simulink model "PlusControllerElegantFix"  (R2021a)
settings: Solver=VariableStepAuto  StartTime=0.0  StopTime=25  RelTol=1e-3
settings Model: Creator=phill  LastModifiedBy=phill

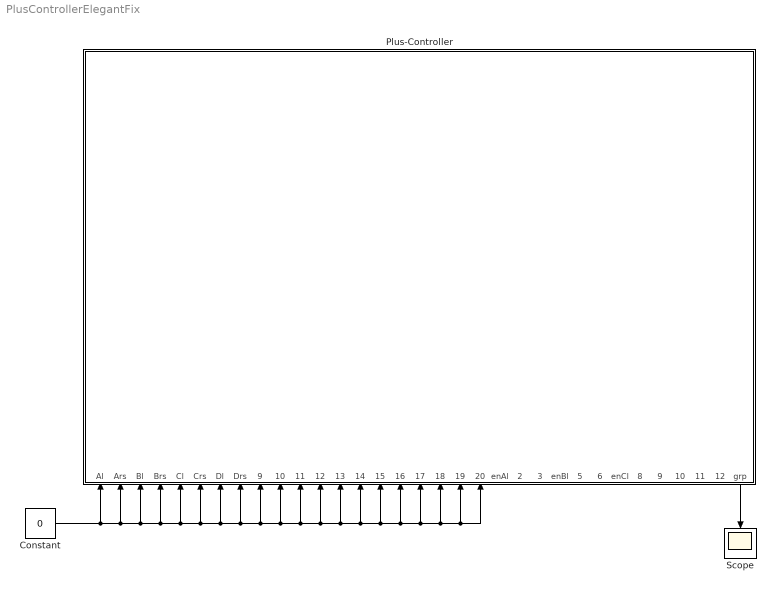
== system PlusControllerElegantFix ==
  Constant : Constant  Value=0
  Plus-Controller : Stateflow chart  TreatAsAtomicUnit=on  mask{green_duration_sr=6, green_duration_l=6, tol=0}
      mask prompts: green_duration_sr "Green Duration for straight/right traffic"; green_duration_l "Green Duration for left traffic"; tol "tolerance"
      settings: PortSchema="{\"entries\":[{\"content\":{\"sides\":[{\"content\":{\"connectorIds\":[]},\"type\":\"ConnectorPlacement.EquallySpacedRectSide\",\"uuid\":\"2590cc03-86a2-4387-8b1b-fdf4c8b68aa6\"},{\"content\":{\"connectorIds\":[],\"side\":\"RIGHT\"},\"type\":\"ConnectorPlacement.EquallySpacedRectSide\",\"uuid\":\"b97063cd-dd31-425f-b4aa-3aaa013ac411\"},{\"content\":{\"connectorIds\":[],\"side\":\"TOP\"},\"type\":\"ConnectorPlacement.EquallySpacedRectSide\",\"uuid\":\"ef5846b9-436e-4b10-a854-1305521b6a0d\"},{\"content\":{\"connectorIds\":[\"In3\",\"In4\",\"In1\",\"In2\",\"In5\",\"In6\",\"In7\",\"In8\",\"In9\",\"In10\",\"In11\",\"In12\",\"In13\",\"In14\",\"In15\",\"In16\",\"In17\",\"In18\",\"In19\",\"In20\",\"Out1\",\"Out2\",\"Out3\",\"Out4\",\"Out5\",\"Out6\",\"Out7\",\"Out8\",\"Out9\",\"Out10\",\"Out11\",\"Out12\",\"Out13\"],\"side\":\"BOTTOM\"},\"type\":\"ConnectorPlacement.EquallySpacedRectSide\",\"uuid\":\"44b73820-3b7c-4ee5-b5da-9465e85a924e\"}]},\"type\":\"ConnectorPlacement.EquallySpacedConnector\",\"uuid\":\"3342797d-7762-4a2a-891a-654024402a66\"}],\"packageUris\":[\"http://schema.mathworks.com/mf0/Connector/R2020b\"],\"version\":\"1.0\"}"
  Scope : Scope
  wires:
  Constant/1 -> Plus-Controller/20(Drs_Bo), Plus-Controller/19(Drs_Ao), Plus-Controller/18(Dl_Co), Plus-Controller/17(Crs_Do), Plus-Controller/16(Crs_Bo), Plus-Controller/15(Cl_Ao), Plus-Controller/14(Brs_Ao), Plus-Controller/13(Brs_Co), Plus-Controller/12(Bl_Do), Plus-Controller/11(Ars_Co), Plus-Controller/10(Ars_Do), Plus-Controller/9(Al_Bo), Plus-Controller/8(Drs), Plus-Controller/7(Dl), Plus-Controller/6(Crs), Plus-Controller/5(Cl), Plus-Controller/2(Brs), Plus-Controller/1(Bl), Plus-Controller/4(Ars), Plus-Controller/3(Al)
  Plus-Controller/13(grp) -> Scope/1

== stateflow chart PlusControllerElegantFix/Plus-Controller ==
  state Group__Crs_Brs
    state init
    note: check
        | Crs straight
        | crossings
    note: check
        | Crs right
        | crossings
    note: check
        | Brs straight
        | crossings
    note: check
        | Brs right
        | crossings
    (default) -> Group__Crs_Brs.init
    (junction 109) -> Group__Crs_Brs.init
    Group__Crs_Brs.init -> (junction 51)
    (junction 51) -> (junction 59) [order 1] : [(Dl_Co<=tol && Drs_Ao<=tol ...
        | && Drs_Bo<=tol && Bl_Do<=tol ...
        | && Al_Bo<=tol && Ars_Do<=tol)]
        | {enCs = 1;}
    (junction 51) -> (junction 59) [order 2] : {enCs = 0;}
    (junction 59) -> (junction 104) [order 1] : [(Ars_Do<=tol && Bl_Do<=tol)]
        | {enCr = 1;}
    (junction 59) -> (junction 104) [order 2] : {enCr = 0;}
    (junction 104) -> (junction 105) [order 1] : [(Al_Bo<=tol && Ars_Do<=tol ...
        | && Ars_Co<=tol && Cl_Ao<=tol ...
        | && Dl_Co<=tol && Drs_Ao<=tol)]
        | {enBs = 1;}
    (junction 104) -> (junction 105) [order 2] : {enBs = 0;}
    (junction 105) -> (junction 109) [order 1] : [Drs_Ao<=tol && Cl_Ao<=tol]
        | {enBr = 1;}
    (junction 105) -> (junction 109) [order 2] : {enBr = 0;}
  state Group__Cl_Bl
    state init
    note: check
        | Cl
        | crossings
    note: check
        | Bl
        | crossings
    (default) -> Group__Cl_Bl.init
    Group__Cl_Bl.init -> (junction 117)
    (junction 126) -> Group__Cl_Bl.init
    (junction 117) -> (junction 116) [order 2] : {enCl = 0;}
    (junction 117) -> (junction 116) [order 1] : [Dl_Co<=tol && Drs_Ao<=tol && ....
        | Brs_Co<=tol && Al_Bo<=tol && ...
        | Ars_Do<=tol && Brs_Ao]{enCl = 1;}
    (junction 116) -> (junction 126) [order 1] : [(Al_Bo<=tol && Ars_Do<=tol && ...
        | Crs_Bo<=tol && Dl_Co<=tol && ...
        | Drs_Ao<=tol && Crs_Do)]{enBl = 1;}
    (junction 116) -> (junction 126) [order 2] : {enBl = 0;}
  state Group__Ars_Drs
    state init
    note: check
        | Ars straight
        | crossings
    note: check
        | Ars right
        | crossings
    note: check
        | Drs straight
        | crossings
    note: check
        | Drs right
        | crossings
    (default) -> Group__Ars_Drs.init
    (junction 131) -> Group__Ars_Drs.init
    Group__Ars_Drs.init -> (junction 134)
    (junction 134) -> (junction 133) [order 1] : [Cl_Ao<=tol && Crs_Bo<=tol && ...
        | Crs_Do<=tol && Dl_Co<=tol && ...
        | Bl_Do<=tol && Brs_Co<=tol]
        | {enAs = 1;}
    (junction 134) -> (junction 133) [order 2] : {enAs = 0;}
    (junction 133) -> (junction 143) [order 1] : [(Brs_Co<=tol && Dl_Co<=tol)]
        | {enAr = 1;}
    (junction 133) -> (junction 143) [order 2] : {enAr = 0;}
    (junction 143) -> (junction 141) [order 1] : [(Bl_Do<=tol && Brs_Co<=tol ...
        | && Brs_Ao<=tol && Al_Bo<=tol ...
        | && Cl_Ao<=tol && Crs_Bo<=tol)]
        | {enDs = 1;}
    (junction 143) -> (junction 141) [order 2] : {enDs=0;}
    (junction 141) -> (junction 131) [order 1] : [(Crs_Bo<=tol && Al_Bo<=tol)]
        | {enDr = 1;}
    (junction 141) -> (junction 131) [order 2] : {enDr = 0;}
  state Group__Al_Dl
    state init
    note: check
        | Al
        | crossings
    note: check
        | Dl
        | crossings
    (default) -> Group__Al_Dl.init
    Group__Al_Dl.init -> (junction 151)
    (junction 160) -> Group__Al_Dl.init
    (junction 151) -> (junction 150) [order 1] : [(Cl_Ao<=tol && Crs_Bo<=tol ...
        | && Drs_Ao<=tol && Bl_Do<=tol ...
        | && Brs_Co<=tol && Drs_Bo)]{enAl = 1;}
    (junction 151) -> (junction 150) [order 2] : {enAl = 0;}
    (junction 150) -> (junction 160) [order 1] : [(Bl_Do<=tol && Brs_Co<=tol ...
        | && Ars_Do<=tol && Cl_Ao<=tol ...
        | && Crs_Bo<=tol && Ars_Co)]{enDl = 1;}
    (junction 150) -> (junction 160) [order 2] : {enDl = 0;}
  Group__Al_Dl -> Group__Crs_Brs : [after(green_duration_l,sec)]
      | {enAl = 0; enDl = 0; grp = 0;}
  Group__Ars_Drs -> Group__Al_Dl : [after(green_duration_sr,sec)]
      | {enAs = 0; enAr = 0; enDs = 0; enDr = 0; grp = grp+1;}
  Group__Cl_Bl -> Group__Ars_Drs : [after(green_duration_l,sec)]
      | {enCl = 0; enBl = 0; grp = grp+1;}
  Group__Crs_Brs -> Group__Cl_Bl : [after(green_duration_sr,sec)]
      | {enCs = 0; enCr = 0; enBs = 0;
      | enBr = 0; grp = grp+1;}
  (default) -> Group__Crs_Brs : {enAl = 0; enAs = 0; enAr = 0;
      | enBl = 0; enBs = 0; enBr = 0;
      | enCl = 0; enCs = 0; enCr = 0;
      | enDl = 0; enDs = 0; enDr = 0;
      | grp = 0;}
  data: Bl input; Brs input; Al input; Ars input; Cl input; Crs input; Dl input; Drs input; Al_Bo input; Ars_Do input; Ars_Co input; Bl_Do input; Brs_Co input; Brs_Ao input; Cl_Ao input; Crs_Bo input; Crs_Do input; Dl_Co input; Drs_Ao input; Drs_Bo input; enAl output =0; enAs output =0; enAr output =0; enBl output =0; enBs output =0; enBr output =0; enCl output =0; enCs output =0; enCr output =0; enDl output =0; enDs output =0; enDr output =0; green_duration_sr parameter; green_duration_l parameter; tol parameter; grp output
